simulink model "bus_accumulator_blk"  (R2019a)
settings: Solver=VariableStepAuto  StartTime=0.0  StopTime=10.0  RelTol=1e-3
libraries: xbsIndex_r4 x6
settings Model: Creator=Ross Donnachie  LastModifiedBy=Ross Donnachie

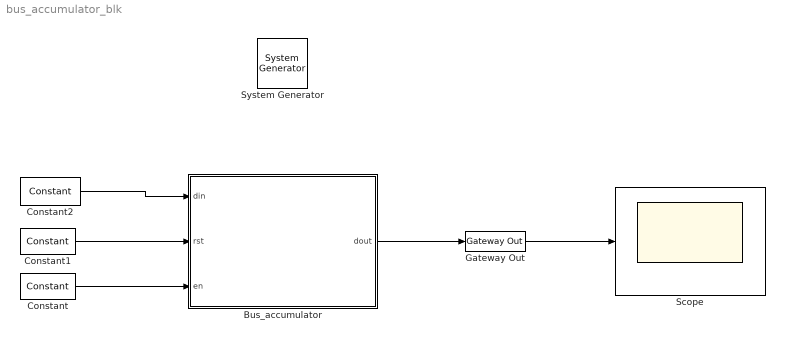
== system bus_accumulator_blk ==
  " System Generator" : xbsIndex_r4/ System Generator  Tag=genX  xilinxfamily=kintex7  part=xc7k325t  speed=-3  package=fbg676  synthesis_tool=Vivado  clock_wrapper=Clock Enables  directory=./netlist  proj_type=Vivado  Synth_file=Vivado Synthesis Defaults  Impl_file=Vivado Implementation Defaults  testbench=off  simulink_period=1  sysclk_period=10  dcm_input_clock_period=10  incr_netlist=off  trim_vbits=Everywhere in SubSystem  dbl_ovrd=According to Block Masks  core_generation=According to Block Masks  run_coregen=off  deprecated_control=off  eval_field=0  block_type=sysgen
  Bus_accumulator : Subsystem  mask{reset_enabled=on, en_enabled=on, input_bit_widths=[4, 8], input_binary_points=[0...], signed=on, complex_input=on, output_bit_widths=[6, 8], overflow_enum=0, misc=off}
      mask prompts: reset_enabled "Reset Port"; en_enabled "Enable Port"; input_bit_widths "Input bit widths"; input_binary_points "Input binary points"; signed "Input type signed (not unsigned)"; complex_input "Complex input (just double bit widths please)"; output_bit_widths "Output bit widths"; overflow_enum "Overflow strategy (Wrap=0, Saturate=1, Flag as error=2)"; misc "Misc support"
      mask init:
      | Simulink.Block.eval([gcb, '/bus_accumulator_stringgenerics']);
      mask DialogControl DescTextVar Prompt: Accumulates the elements in the bus.
      mask DialogControl Control2 Prompt: Pluralised fields are '[]' encapsulated, comma-separated lists.
  Constant : xbsIndex_r4/Constant  const=1  gui_display_data_type=Boolean  arith_type=Boolean  n_bits=16  bin_pt=14  preci_type=Single  exp_width=8  frac_width=24  explicit_period=on  period=1  equ=P=C  opselect=C  inp2=PCIN>>17  opr=+  inp1=P  carry=CIN  dbl_ovrd=off  block_type=constant
  Constant1 : xbsIndex_r4/Constant  const=0  gui_display_data_type=Boolean  arith_type=Boolean  n_bits=16  bin_pt=14  preci_type=Single  exp_width=8  frac_width=24  explicit_period=on  period=1  equ=P=C  opselect=C  inp2=PCIN>>17  opr=+  inp1=P  carry=CIN  dbl_ovrd=off  block_type=constant
  Constant2 : xbsIndex_r4/Constant  const=257  gui_display_data_type=Fixed-point  arith_type=Signed (2's comp)  n_bits=12  bin_pt=0  preci_type=Single  exp_width=8  frac_width=24  explicit_period=on  period=1  equ=P=C  opselect=C  inp2=PCIN>>17  opr=+  inp1=P  carry=CIN  dbl_ovrd=off  block_type=constant
  Gateway Out : xbsIndex_r4/Gateway Out  inherit_from_input=on  hdl_port=on  rows=1  columns=1  UseAsDAC=off  DACChannel='1'  interface=None  automatic_assignment=on  address_offset=hex2dec('00')  intf_name=''  intf_description=''  timing_constraint=None  locs_specified=off  LOCs={}  io_standard={}  block_type=gatewayout
  Scope : Scope
  wires:
  Constant/1 -> Bus_accumulator/3(en)
  Constant1/1 -> Bus_accumulator/2(rst)
  Constant2/1 -> Bus_accumulator/1(din)
  Bus_accumulator/1(dout) -> Gateway Out/1
  Gateway Out/1 -> Scope/1

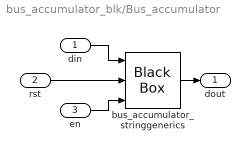
== system bus_accumulator_blk/Bus_accumulator ==
  din : Inport
  rst : Inport  Port=2
  en : Inport  Port=3
  bus_accumulator_stringgenerics : xbsIndex_r4/Black Box  init_code=bus_accumulator_stringgenerics_config  sim_method=ISE Simulator  verbose=off  block_type=blackbox2
  dout : Outport
  wires:
  en/1 -> bus_accumulator_stringgenerics/3
  din/1 -> bus_accumulator_stringgenerics/1
  bus_accumulator_stringgenerics/1 -> dout/1
  rst/1 -> bus_accumulator_stringgenerics/2
